simulink model "Bloque_calentamiento"  (R2022b)
settings: Solver=VariableStepAuto  StartTime=0.0  StopTime=5  RelTol=1e-3
undefined symbols (not defined in the file or in its folder): magnitude
settings Model: Creator=Javier  LastModifiedBy=mique
settings DebuggingCC: UnconnectedInputMsg=warning  UnconnectedOutputMsg=warning  UnconnectedLineMsg=warning
settings ModelReferenceCC: EnableRefExpFcnMdlSchedulingChecks=on
settings RTWCC: DLArmComputeVersion=19.05

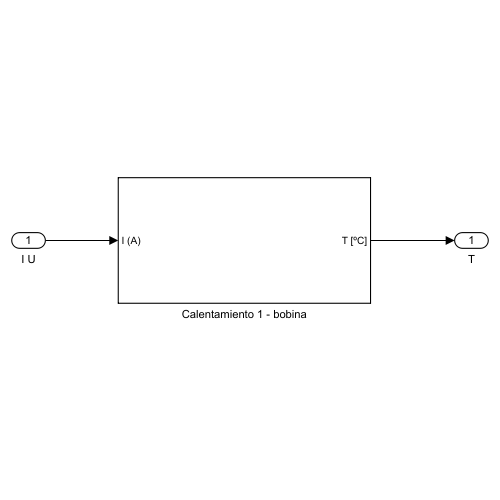
[thumbnail: Simulink's stored preview of the top-level diagram]
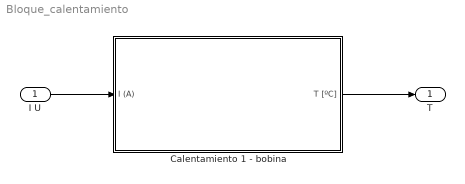
== system Bloque_calentamiento ==
  I U : Inport
  Calentamiento 1 - bobina : Subsystem
  T : Outport
  wires:
  Calentamiento 1 - bobina/1(T [ºC]) -> T/1
  I U/1 -> Calentamiento 1 - bobina/1(I (A))

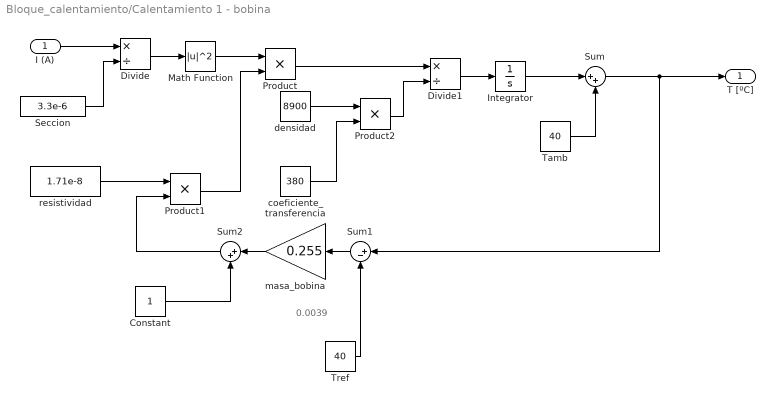
== system Bloque_calentamiento/Calentamiento 1 - bobina ==
  note: 0.0039
  I (A) : Inport
  Constant : Constant
  Divide : Product  Inputs=*/
  Divide1 : Product  Inputs=*/
  Integrator : Integrator
  Math Function : Math  Operator=magnitude^2
  Product : Product
  Product1 : Product
  Product2 : Product
  Seccion : Constant  Value=3.3e-6
  Sum : Sum  Inputs=|++
  Sum1 : Sum  Inputs=|+-
  Sum2 : Sum  Inputs=|++
  Tamb : Constant  Value=40
  Tref : Constant  Value=40
  coeficiente_transferencia : Constant  Value=380
  densidad : Constant  Value=8900
  masa_bobina : Gain  Gain=0.255
  resistividad : Constant  Value=1.71e-8
  T [ºC] : Outport
  wires:
  I (A)/1 -> Divide/1
  Seccion/1 -> Divide/2
  Divide/1 -> Math Function/1
  Math Function/1 -> Product/1
  Product/1 -> Divide1/1
  Divide1/1 -> Integrator/1
  Integrator/1 -> Sum/1
  Tamb/1 -> Sum/2
  Sum/1 -> Sum1/1, T [ºC]/1
  Sum1/1 -> masa_bobina/1
  Tref/1 -> Sum1/2
  masa_bobina/1 -> Sum2/1
  Constant/1 -> Sum2/2
  resistividad/1 -> Product1/1
  Sum2/1 -> Product1/2
  Product1/1 -> Product/2
  Product2/1 -> Divide1/2
  densidad/1 -> Product2/1
  coeficiente_transferencia/1 -> Product2/2
